simulink model "TDE_with_NPD_ARAS"  (R2018b)
settings: Solver=FixedStepAuto  StartTime=0.0  StopTime=24.5  FixedStep=.001  RelTol=1e-3
settings Model: Creator=ahmad  LastModifiedBy=asus
settings SFSimCC: SimUseLocalCustomCode=off
settings RTWCC: RTWUseLocalCustomCode=off
settings CodeAppCC: StateflowObjectComments=on

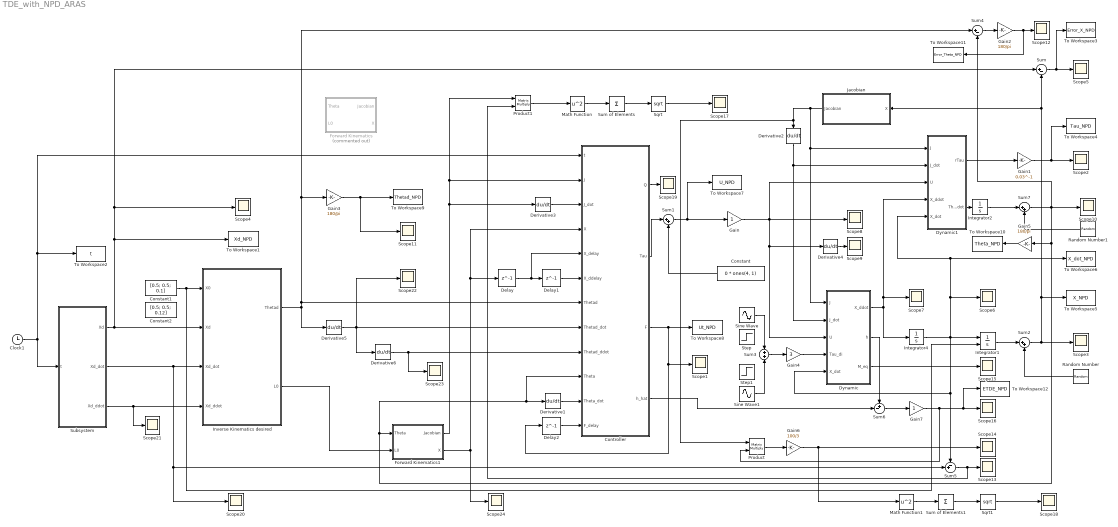
== system TDE_with_NPD_ARAS ==
  Clock1 : Clock
  Constant : Constant  Value=0 * ones(4, 1)
  Constant1 : Constant  Value=[0.5; 0.5; 0.1]
  Constant2 : Constant  Value=[0.5; 0.5; 0.12]
  "Controller " : MATLAB Function  TreatAsAtomicUnit=on
  Delay : Delay  DelayLength=1  InitialCondition=[0; 0; 0]
  Delay1 : Delay  DelayLength=1  InitialCondition=[0; 0; 0]
  Delay2 : Delay  DelayLength=1  InitialCondition=[0; 0; 0]
  Derivative{1..6} (6 alike) : Derivative
  Dynamic : MATLAB Function  TreatAsAtomicUnit=on
  Dynamic1 : MATLAB Function  TreatAsAtomicUnit=on
  Forward Kinematics : MATLAB Function  Commented=on  TreatAsAtomicUnit=on
  Forward Kinematics1 : MATLAB Function  TreatAsAtomicUnit=on
  Gain : Gain
  Gain1 : Gain  Gain=0.03^-1
  Gain2 : Gain  Gain=180/pi
  Gain3 : Gain  Gain=180/pi
  Gain4 : Gain  Gain=3
  Gain5 : Gain  Gain=180/pi
  Gain6 : Gain  Gain=100/3
  Gain7 : Gain
  Integrator1 : Integrator  InitialConditionSource=external  InitialCondition=[0.5; 0.5; 0.5]
  Integrator2 : Integrator  InitialCondition=[0;0;0;0]
  Integrator4 : Integrator  InitialCondition=[0;0;0]
  Inverse Kinematics desired : MATLAB Function  TreatAsAtomicUnit=on
  Jacobian : MATLAB Function  TreatAsAtomicUnit=on
  Math Function : Math  Operator=square  SaturateOnIntegerOverflow=on
  Math Function1 : Math  Operator=square  SaturateOnIntegerOverflow=on
  Product : Product  Multiplication=Matrix(*)
  Product1 : Product  Multiplication=Matrix(*)
  Random Number : RandomNumber  Mean=[0;0;0]  Variance=0.0000 * ones(3, 1)  SampleTime=0.01
  Random Number1 : RandomNumber  Mean=[0;0;0;0]  Variance=0.0000 * ones(4, 1)  SampleTime=0.01
  Scope{1..24} (24 alike) : Scope
  Sine Wave : Sin  Phase=pi/2
  Sine Wave1 : Sin  Amplitude=0
  Sqrt : Sqrt  SaturateOnIntegerOverflow=on
  Sqrt1 : Sqrt  SaturateOnIntegerOverflow=on
  Step : Step  Time=15  Before=[0; 0; 0]  After=[-1; 1; 1]  SampleTime=0.001
  Step1 : Step  Time=17  Before=[0; 0; 0]  After=[1; -1; -1]  SampleTime=0.001
  Subsystem : Subsystem
  Sum : Sum  Inputs=|+-
  Sum of Elements : Sum  Inputs=+
  Sum of Elements1 : Sum  Inputs=+
  Sum1 : Sum  Inputs=|++
  Sum2 : Sum  Inputs=|++
  Sum3 : Sum
  Sum4 : Sum  Inputs=|+-
  Sum5 : Sum  Inputs=-+|
  Sum6 : Sum  Inputs=+-|
  Sum7 : Sum  Inputs=|++
  To Workspace1 : ToWorkspace  VariableName=Xd_NPD  SampleTime=-1
  To Workspace10 : ToWorkspace  VariableName=Theta_NPD  SampleTime=-1
  To Workspace11 : ToWorkspace  VariableName=Error_Theta_NPD  SampleTime=-1
  To Workspace12 : ToWorkspace  VariableName=ETDE_NPD  SampleTime=-1
  To Workspace2 : ToWorkspace  VariableName=t  SampleTime=-1
  To Workspace3 : ToWorkspace  VariableName=Error_X_NPD  SampleTime=-1
  To Workspace4 : ToWorkspace  VariableName=Tau_NPD  SampleTime=-1
  To Workspace5 : ToWorkspace  VariableName=X_NPD  SampleTime=-1
  To Workspace6 : ToWorkspace  VariableName=X_dot_NPD  SampleTime=-1
  To Workspace7 : ToWorkspace  VariableName=U_NPD  SampleTime=-1
  To Workspace8 : ToWorkspace  VariableName=Ut_NPD  SampleTime=-1
  To Workspace9 : ToWorkspace  VariableName=Thetad_NPD  SampleTime=-1
  wires:
  Integrator1/1 -> Sum2/1
  Sum/1 -> To Workspace3/1, Scope5/1
  Constant/1 -> Sum1/2
  Random Number/1 -> Sum2/2
  Sum2/1 -> To Workspace5/1, Jacobian/1(X), Sum/2, Scope3/1
  Clock1/1 -> To Workspace2/1, "Controller "/1(t), Subsystem/1(t)
  Delay/1 -> "Controller "/5(X_delay), Delay1/1
  Delay1/1 -> "Controller "/6(X_ddelay)
  "Controller "/3(F) -> Delay2/1, Scope1/1, To Workspace8/1
  "Controller "/2(Tau) -> Sum1/1
  Delay2/1 -> "Controller "/12(F_delay)
  Sum1/1 -> Gain/1, To Workspace7/1
  Inverse Kinematics desired/1(Thetad) -> Derivative5/1, Gain3/1, Sum4/1, "Controller "/7(Thetad)
  Derivative1/1 -> "Controller "/11(Theta_dot)
  Sum3/1 -> Gain4/1
  Sine Wave/1 -> Sum3/1
  Sine Wave1/1 -> Sum3/2
  Gain1/1 -> To Workspace4/1, Scope2/1
  Dynamic/1(X_ddot) -> Integrator4/1, Dynamic1/4(X_ddot), Scope7/1
  Jacobian/1(Jacobian) -> Product/1, Derivative2/1, Dynamic1/1(J), Dynamic/1(J)
  Derivative3/1 -> "Controller "/3(J_dot)
  Integrator4/1 -> To Workspace6/1, Dynamic1/5(X_dot), Scope6/1, Sum5/1, Dynamic/5(X_dot), Integrator1/1
  Dynamic1/1(rTau) -> Gain1/1
  Gain/1 -> Derivative4/1, Dynamic/3(U), Scope8/1, Dynamic1/3(U)
  Forward Kinematics1/1(Jacobian) -> Product1/1, "Controller "/2(J), Derivative3/1
  Forward Kinematics1/2(X) -> "Controller "/4(X), Delay/1, Scope24/1
  Derivative2/1 -> Dynamic/2(J_dot), Dynamic1/2(J_dot)
  Subsystem/1(Xd) -> Inverse Kinematics desired/2(Xd), To Workspace1/1, Scope4/1, Sum/1
  Subsystem/2(Xd_dot) -> Scope20/1, Sum5/2, Inverse Kinematics desired/3(Xd_dot)
  Subsystem/3(Xd_ddot) -> Scope21/1, Inverse Kinematics desired/4(Xd_ddot)
  Derivative4/1 -> Scope9/1
  Dynamic1/2(Theta_dot) -> Integrator2/1
  Sum7/1 -> Sum4/2, Forward Kinematics1/1(Theta), "Controller "/10(Theta), Derivative1/1, Gain5/1, Scope10/1
  Sum4/1 -> Gain2/1
  Gain2/1 -> To Workspace11/1, Scope12/1
  Gain3/1 -> Scope11/1, To Workspace9/1
  Gain4/1 -> Dynamic/4(Tau_di)
  Gain5/1 -> To Workspace10/1
  Dynamic/2(h) -> Sum6/1
  "Controller "/4(h_hat) -> Sum6/2
  Sum6/1 -> Gain7/1
  Product/1 -> Gain6/1
  Dynamic/3(M_eq) -> Scope15/1
  Sum of Elements/1 -> Sqrt/1
  Math Function/1 -> Sum of Elements/1
  Sum5/1 -> Product1/2, Scope13/1
  Product1/1 -> Math Function/1
  Sqrt/1 -> Scope17/1
  Gain6/1 -> Math Function1/1, Scope14/1
  Sqrt1/1 -> Scope18/1
  Math Function1/1 -> Sum of Elements1/1
  Sum of Elements1/1 -> Sqrt1/1
  Integrator2/1 -> Sum7/1
  Random Number1/1 -> Sum7/2
  "Controller "/1(Q) -> Scope19/1
  Constant1/1 -> Inverse Kinematics desired/1(X0), Integrator1/2
  Derivative5/1 -> Derivative6/1, Scope22/1, "Controller "/8(Thetad_dot)
  Derivative6/1 -> Scope23/1, "Controller "/9(Thetad_ddot)
  Inverse Kinematics desired/2(L0) -> Forward Kinematics1/2(L0)
  Gain7/1 -> Product/2, To Workspace12/1, Scope16/1

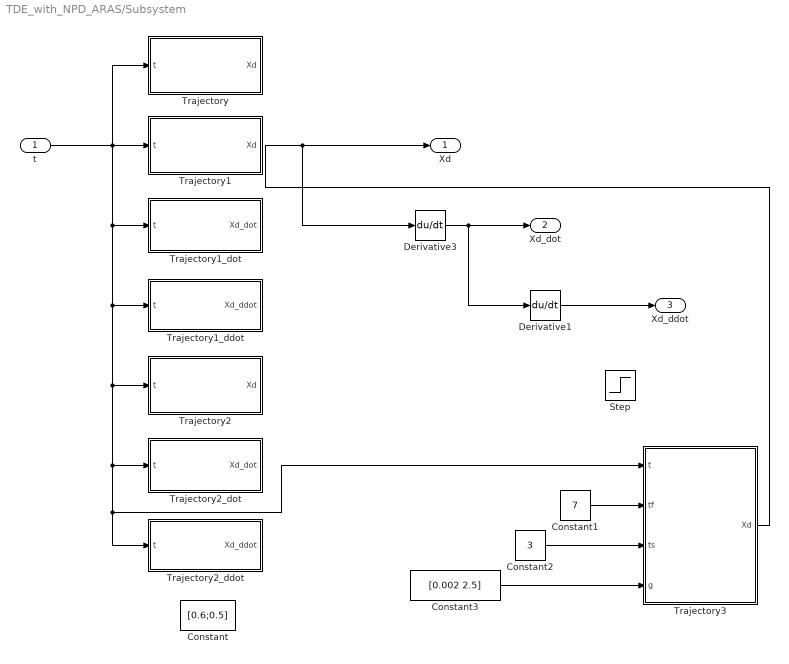
== system TDE_with_NPD_ARAS/Subsystem ==
  t : Inport
  Constant : Constant  Value=[0.6;0.5]
  Constant1 : Constant  Value=7
  Constant2 : Constant  Value=3
  Constant3 : Constant  Value=[0.002 2.5]
  Derivative1 : Derivative
  Derivative3 : Derivative
  Step : Step  Time=10  Before=[0.5; 0.5; 0.1]  After=[0.5; 0.5; 0.13]  SampleTime=0.001
  Trajectory : MATLAB Function  TreatAsAtomicUnit=on
  Trajectory1 : MATLAB Function  TreatAsAtomicUnit=on
  Trajectory1_ddot : MATLAB Function  TreatAsAtomicUnit=on
  Trajectory1_dot : MATLAB Function  TreatAsAtomicUnit=on
  Trajectory2 : MATLAB Function  TreatAsAtomicUnit=on
  Trajectory2_ddot : MATLAB Function  TreatAsAtomicUnit=on
  Trajectory2_dot : MATLAB Function  TreatAsAtomicUnit=on
  Trajectory3 : MATLAB Function  TreatAsAtomicUnit=on
  Xd : Outport
  Xd_dot : Outport  Port=2
  Xd_ddot : Outport  Port=3
  wires:
  Trajectory3/1(Xd) -> Derivative3/1, Xd/1
  Derivative3/1 -> Derivative1/1, Xd_dot/1
  Derivative1/1 -> Xd_ddot/1
  Constant2/1 -> Trajectory3/3(ts)
  Constant3/1 -> Trajectory3/4(g)
  Constant1/1 -> Trajectory3/2(tf)
  t/1 -> Trajectory/1(t), Trajectory3/1(t), Trajectory2_ddot/1(t), Trajectory2_dot/1(t), Trajectory2/1(t), Trajectory1_ddot/1(t), Trajectory1_dot/1(t), Trajectory1/1(t)

== matlab function TDE_with_NPD_ARAS/Dynamic ==
  data: J input; J_dot input; U input; Tau_di input; X_ddot output; X_dot input; h output; M_eq output
function [X_ddot, h, M_eq] = fcn(J, J_dot, U, Tau_di, X_dot)

M_bar = 0.01 * eye(3);
m = 1.5;
g = 9.81;
r = 0.03;

Im = 8.31 * 10^-5 * eye(4);
Dm = 2.16 * 10^-4 * eye(4);

M = m * eye(3);
C = zeros(3, 3);
G = [0; 0; m*g];
N = C * X_dot + G + 0.5 * sign(X_dot) + 0.5 * X_dot + Tau_di;

M_eq = r * M + r^-1 * J' * Im * J;
N_eq = r * N + r^-1 * J' * Im * J_dot * X_dot + r^-1 * J' * Dm * J * X_dot;
% W = J';
Tau = J' * U;
X_ddot = M_eq^(-1) * (Tau - N_eq);
h = (M_eq - M_bar) * X_ddot + N_eq;
end

== matlab function TDE_with_NPD_ARAS/Dynamic1 ==
  data: J input; rTau output; J_dot input; U input; X_ddot input; X_dot input; Theta_dot output
function [rTau, Theta_dot] = fcn(J, J_dot, U, X_ddot, X_dot)

r = 0.03;
Im = 8.31 * 10^-5 * eye(4);
Dm = 2.16 * 10^-4 * eye(4);

Theta_dot = r^-1 * J * X_dot;
Theta_ddot = r^-1 * (J * X_ddot + J_dot * X_dot);

rTau = Im * Theta_ddot + Dm * Theta_dot - U;
end

== matlab function TDE_with_NPD_ARAS/Subsystem/Trajectory1 ==
  data: Xd output; t input
function Xd = fcn(t)

a = 1.00;
b = 1.00;
r = 0.1;
f = 0.5;

x = r * (cos(2*pi*f*t)) + a/2;
y = r * (sin(2*pi*f*t)) + b/2;

Xd = [x y]';
end

== matlab function TDE_with_NPD_ARAS/Inverse Kinematics desired ==
  data: X0 input; Xd input; Thetad output; Xd_dot input; Xd_ddot input; L0 output
function [Thetad, L0]  = fcn(X0, Xd, Xd_dot, Xd_ddot)

a = 1.00;% + 0.05;
b = 1.00;% - 0.05;
c = 1.00;% - 0.05;
r = 0.03;

% A1 = [0+0.02 0-0.01 c-0.1]';
% A2 = [0+0.01 b+0.01 c+0.1]';
% A3 = [a-0.02 b-0.02 c-0.02]';
% A4 = [a-0.01 0+0.02 c+0.02]';
A1 = [0 0 c]';
A2 = [0 b c]';
A3 = [a b c]';
A4 = [a 0 c]';

L0 = [sqrt((X0(1)-A1(1))^2 + (X0(2)-A1(2))^2 + (X0(3)-A1(3))^2)
      sqrt((X0(1)-A2(1))^2 + (X0(2)-A2(2))^2 + (X0(3)-A2(3))^2)
      sqrt((X0(1)-A3(1))^2 + (X0(2)-A3(2))^2 + (X0(3)-A3(3))^2)
      sqrt((X0(1)-A4(1))^2 + (X0(2)-A4(2))^2 + (X0(3)-A4(3))^2)];

L = [sqrt((Xd(1)-A1(1))^2 + (Xd(2)-A1(2))^2 + (Xd(3)-A1(3))^2)
     sqrt((Xd(1)-A2(1))^2 + (Xd(2)-A2(2))^2 + (Xd(3)-A2(3))^2)
     sqrt((Xd(1)-A3(1))^2 + (Xd(2)-A3(2))^2 + (Xd(3)-A3(3))^2)
     sqrt((Xd(1)-A4(1))^2 + (Xd(2)-A4(2))^2 + (Xd(3)-A4(3))^2)];
 
Thetad = r^-1 * (L - L0);
end

== matlab function TDE_with_NPD_ARAS/Forward Kinematics ==
  data: Jacobian output; Theta input; X output; L0 input
function [Jacobian, X] = fcn(Theta, L0)

a = 1.00;% + 0.05;
b = 1.00;% - 0.05;
c = 1.00;% - 0.05;
r = 0.03;% + 0.005;

A1 = [0 0 c]';
A2 = [0 b c]';
A3 = [a b c]';
A4 = [a 0 c]';
% A1 = [0+0.02 0-0.01 c-0.1]';
% A2 = [0+0.01 b+0.01 c+0.1]';
% A3 = [a-0.02 b-0.02 c-0.02]';
% A4 = [a-0.01 0+0.02 c+0.02]';

L = [r * Theta(1) + L0(1)
     r * Theta(2) + L0(2)
     r * Theta(3) + L0(3)
     r * Theta(4) + L0(4)];
% dgfd
g1 = A1(1)^2-A2(1)^2+A1(2)^2-A2(2)^2+A1(3)^2-A2(3)^2;
g2 = A1(1)^2-A3(1)^2+A1(2)^2-A3(2)^2+A1(3)^2-A3(3)^2;

e1 = (L(1)^2-L(2)^2-g1) / (2*(A2(2)-A1(2)));
e2 = (A2(1)-A1(1)) / (A2(2)-A1(2));
e3 = (A2(3)*A1(3)) / (A2(2)-A1(2));
f1 = (L(1)^2-L(3)^2-g2) / (2*(A3(1)-A1(1)));
f2 = (A3(2)-A1(2)) / (A3(1)-A1(1));
f3 = (A3(3)-A1(3)) / (A3(1)-A1(1));

d1 = (e1-e2*f1) / (1-e2*f2);
d2 = (e3-e2*f3) / (1-e2*f2);
d3 = f1-f2*d1;
d4 = f2*d2-f3;

A = 1 + d2^2 + d4^2;
B = 2*(d3*d4-A1(1)*d4-d1*d2+A1(2)*d2-A1(3));
C = d3^2+A1(1)^2-2*A1(1)*d3+d1^2+A1(2)^2-2*A1(2)*d1+A1(3)^2-L(1)^2;

z = (-B-sqrt(B^2-4*A*C)) / (2*A);
y = d1 - d2 * z;
x = d3 + d4 * z;
% x = (L(2)^2 - L(3)^2 + a^2) / (2*a);
% y = (L(1)^2 - L(2)^2 + b^2) / (2*b);
% z = c - sqrt(L(1)^2 - x^2 - y^2);
X = [x y z]';

Jacobian = [(X(1)-A1(1))/L(1)    (X(2)-A1(2))/L(1)   (X(3)-A1(3))/L(1)
            (X(1)-A2(1))/L(2)    (X(2)-A2(2))/L(2)   (X(3)-A2(3))/L(2)
            (X(1)-A3(1))/L(3)    (X(2)-A3(2))/L(3)   (X(3)-A3(3))/L(3)
            (X(1)-A4(1))/L(4)    (X(2)-A4(2))/L(4)   (X(3)-A4(3))/L(4)];
end

== matlab function TDE_with_NPD_ARAS/Subsystem/Trajectory ==
  data: Xd output; t input
function Xd  = fcn(t)

a = 1.00;
b = 1.00;
ts = 2;
tf = 5;

if t <= ts
    x0 = a / 2;
    y0 = b / 2;
    Xd = [x0 y0]';
elseif t > ts && t < tf+ts
    x0 = a / 2; xf = x0 - 0.0; x_dot0 = 0; x_dotf = 0; x_ddot0 = 0; x_ddotf = 0;
    a0 = x0; a1 = x_dot0; a2 = x_ddot0 / 2;
    a3 = (20*(xf-x0)-(8*x_dotf+12*x_dot0)*tf-(3*x_ddot0-x_ddotf)*tf^2) / (2*tf^3);
    a4 = (30*(x0-xf)+(14*x_dotf+16*x_dot0)*tf+(3*x_ddot0-2*x_ddotf)*tf^2) / (2*tf^4);
    a5 = (12*(xf-x0)-(6*x_dotf+6*x_dot0)*tf-(x_ddot0-x_ddotf)*tf^2) / (2*tf^5);
    x = a0 + a1 * (t-ts) + a2 * (t-ts)^2 + a3 * (t-ts)^3 + a4 * (t-ts)^4 + a5 * (t-ts)^5;
    
    y0 = b / 2; yf = y0 + 0.2; y_dot0 = 0; y_dotf = 0; y_ddot0 = 0; y_ddotf = 0;
    b0 = y0; b1 = y_dot0; b2 = y_ddot0 / 2;
    b3 = (20*(yf-y0)-(8*y_dotf+12*y_dot0)*tf-(3*y_ddot0-y_ddotf)*tf^2) / (2*tf^3);
    b4 = (30*(y0-yf)+(14*y_dotf+16*y_dot0)*tf+(3*y_ddot0-2*y_ddotf)*tf^2) / (2*tf^4);
    b5 = (12*(yf-y0)-(6*y_dotf+6*y_dot0)*tf-(y_ddot0-y_ddotf)*tf^2) / (2*tf^5);
    y = b0 + b1 * (t-ts) + b2 * (t-ts)^2 + b3 * (t-ts)^3 + b4 * (t-ts)^4 + b5 * (t-ts)^5;
    
    Xd = [x y]';
elseif t >= tf+ts && t < 10
    x0 = a / 2; xf = x0 - 0.0;
    y0 = b / 2; yf = y0 + 0.2;
    
    Xd = [xf yf]';
elseif t >= 10 && t < 30
    f = 0.05;
    x = 0.5 + 0.2*sin(2*pi*f*(t-10));
    y = 0.5 + 0.2*cos(2*pi*f*(t-10));

    Xd = [x y]';
elseif t >= 30 && t < 40
    f = 0.1;
    x = 0.5 + 0.2*sin(2*pi*f*(t-30));
    y = 0.5 + 0.2*cos(2*pi*f*(t-30));

    Xd = [x y]';
elseif t >= 40 && t < 45
    f = 0.2;
    x = 0.5 + 0.2*sin(2*pi*f*(t-40));
    y = 0.5 + 0.2*cos(2*pi*f*(t-40));

    Xd = [x y]';
elseif t >= 45 && t < 47
    f = 0.5;
    x = 0.5 + 0.2*sin(2*pi*f*(t-45));
    y = 0.5 + 0.2*cos(2*pi*f*(t-45));

    Xd = [x y]';
elseif t >= 47 && t < 49
    f = 0.5;
    x = 0.5 + 0.2*sin(2*pi*f*(t-47));
    y = 0.5 + 0.2*cos(2*pi*f*(t-47));

    Xd = [x y]';
elseif t >= 49 && t < 54
    f = 0.2;
    x = 0.5 + 0.2*sin(2*pi*f*(t-49));
    y = 0.5 + 0.2*cos(2*pi*f*(t-49));

    Xd = [x y]';
elseif t >= 54 && t < 64
    f = 0.1;
    x = 0.5 + 0.2*sin(2*pi*f*(t-54));
    y = 0.5 + 0.2*cos(2*pi*f*(t-54));

    Xd = [x y]';
elseif t >= 64 && t < 84
    f = 0.05;
    x = 0.5 + 0.2*sin(2*pi*f*(t-64));
    y = 0.5 + 0.2*cos(2*pi*f*(t-64));

    Xd = [x y]';
elseif t >= 84 && t < tf+84
    x0 = a / 2; xf = x0 - 0.0; x_dot0 = 0; x_dotf = 0; x_ddot0 = 0; x_ddotf = 0;
    a0 = x0; a1 = x_dot0; a2 = x_ddot0 / 2;
    a3 = (20*(xf-x0)-(8*x_dotf+12*x_dot0)*tf-(3*x_ddot0-x_ddotf)*tf^2) / (2*tf^3);
    a4 = (30*(x0-xf)+(14*x_dotf+16*x_dot0)*tf+(3*x_ddot0-2*x_ddotf)*tf^2) / (2*tf^4);
    a5 = (12*(xf-x0)-(6*x_dotf+6*x_dot0)*tf-(x_ddot0-x_ddotf)*tf^2) / (2*tf^5);
    x = a0 + a1 * (t-84) + a2 * (t-84)^2 + a3 * (t-84)^3 + a4 * (t-84)^4 + a5 * (t-84)^5;
    
    y0 = b / 2 + 0.2; yf = y0 - 0.2; y_dot0 = 0; y_dotf = 0; y_ddot0 = 0; y_ddotf = 0;
    b0 = y0; b1 = y_dot0; b2 = y_ddot0 / 2;
    b3 = (20*(yf-y0)-(8*y_dotf+12*y_dot0)*tf-(3*y_ddot0-y_ddotf)*tf^2) / (2*tf^3);
    b4 = (30*(y0-yf)+(14*y_dotf+16*y_dot0)*tf+(3*y_ddot0-2*y_ddotf)*tf^2) / (2*tf^4);
    b5 = (12*(yf-y0)-(6*y_dotf+6*y_dot0)*tf-(y_ddot0-y_ddotf)*tf^2) / (2*tf^5);
    y = b0 + b1 * (t-84) + b2 * (t-84)^2 + b3 * (t-84)^3 + b4 * (t-84)^4 + b5 * (t-84)^5;
    
    Xd = [x y]';
else
    x0 = a / 2;
    y0 = b / 2;
    xf = x0 + 0.0;
    yf = y0 + 0.0;
    Xd = [xf yf]';
end

end

== matlab function TDE_with_NPD_ARAS/Subsystem/Trajectory2 ==
  data: Xd output; t input
function Xd = fcn(t)

T = 0.001;
a = 1;
b = 1;

x0 = b / 2 - 0.1; xf = x0 + 0.3; x_dot0 = 0; x_dotf = 0; tf = 10;
a0 = x0; a1 = x_dot0; a2 = (3/tf^2) * (xf-x0) - ((x_dotf+2*x_dot0) / tf); a3 = (-2/tf^3) * (xf-x0) + (x_dotf+x_dot0) / tf^2;
x = a0 + a1 * t + a2 * t^2 + a3 * t^3;
x_new = a0 + a1 * (t + T) + a2 * (t + T)^2 + a3 * (t + T)^3;

y0 = a / 2 - 0.1; yf = y0 + 0.3; y_dot0 = 0; y_dotf = 0;
b0 = y0; b1 = y_dot0; b2 = (3/tf^2) * (yf-y0) - ((y_dotf+2*y_dot0) / tf); b3 = (-2/tf^3) * (yf-y0) + (y_dotf+y_dot0) / tf^2;
y = b0 + b1 * t + b2 * t^2 + b3 * t^3;
y_new = b0 + b1 * (t + T) + b2 * (t + T)^2 + b3 * (t + T)^3;

Xd = [x y]';
Xr_new = [x_new y_new]';
end

== matlab function TDE_with_NPD_ARAS/Jacobian ==
  data: Jacobian output; X input
function Jacobian = fcn(X)

a = 1.00;
b = 1.00;
c = 1.00;
% r = 0.03;

L = [sqrt((X(1)-0)^2 + (X(2)-0)^2 + (X(3)-c)^2)
     sqrt((X(1)-0)^2 + (X(2)-b)^2 + (X(3)-c)^2)
     sqrt((X(1)-a)^2 + (X(2)-b)^2 + (X(3)-c)^2)
     sqrt((X(1)-a)^2 + (X(2)-0)^2 + (X(3)-c)^2)];

Jacobian = [(X(1)-0)/L(1)    (X(2)-0)/L(1)   (X(3)-c)/L(1)
            (X(1)-0)/L(2)    (X(2)-b)/L(2)   (X(3)-c)/L(2)
            (X(1)-a)/L(3)    (X(2)-b)/L(3)   (X(3)-c)/L(3)
            (X(1)-a)/L(4)    (X(2)-0)/L(4)   (X(3)-c)/L(4)];
end

== matlab function TDE_with_NPD_ARAS/Controller  ==
  settings: updateMethod=DISCRETE
  data: Q output; t input; Tau output; J input; J_dot input; X input; X_delay input; X_ddelay input; Thetad input; Thetad_dot input; Thetad_ddot input; Theta input; Theta_dot input; F_delay input; F output; h_hat output
function [Q, Tau, F, h_hat] = fcn(t, J, J_dot, X, X_delay, X_ddelay, Thetad, Thetad_dot, Thetad_ddot, Theta, Theta_dot, F_delay)

T = 0.001;
r = 0.03 ;%+ 0.005;
Q = zeros(4, 1);
k = -2;
% tau_min = [0.01 0.01 0.01]';
% tau_max = [1.5 1.5 1.5]';

deltap = 5 * 10^-4;
deltav = 5 * 10^-4;
alphap = 0.3;
alphav = 1.4;
M_bar = 0.01 * eye(3);
Kp = 25 * eye(4);
Kv = 2 * Kp.^0.5;
Ke = 10 * eye(4);

Error = Thetad - Theta;
Error_dot = Thetad_dot - Theta_dot;

if norm(Error) > deltap
    N_Kp = Kp * diag((abs(Error)).^(alphap - 1));
else
    N_Kp = diag([deltap.^(alphap - 1), deltap.^(alphap - 1), deltap.^(alphap - 1), deltap.^(alphap - 1)]);
end

if norm(Error_dot) > deltav
    N_Kv = Kv * diag((abs(Error_dot)).^(alphav - 1));
else
    N_Kv = diag([deltav.^(alphav - 1), deltav.^(alphav - 1), deltav.^(alphav - 1), deltav.^(alphav - 1)]);
end

if t <= 2*T
    X_ddot_delay = zeros(3, 1);
else
    X_ddot_delay = (X - 2 * X_delay + X_ddelay) / T^2;
end

h_hat = F_delay - M_bar * X_ddot_delay;

W = J';
Ur = M_bar * (r * pinv(J) * (Thetad_ddot + N_Kv * Error_dot + N_Kp * Error - J_dot * pinv(J) * Theta_dot + Ke * sat(Error_dot))) + h_hat;
Tau = pinv(W) * Ur; % + k * null(W);
Q = pinv(W) * Ur + k * null(W) - pinv(W) * Ur;
F = W * Tau;
end

function S = sat(E_dot)

varpi = 0.10;

if norm(E_dot) >= varpi
     S = E_dot / norm(E_dot);
else
    S = E_dot / varpi;
end
end

== matlab function TDE_with_NPD_ARAS/Subsystem/Trajectory1_ddot ==
  data: Xd_ddot output; t input
function Xd_ddot = fcn(t)

a = 1.00;
b = 1.00;
r = 0.1;
f = 0.5;

x_ddot = -r * ((2*pi*f)^2*cos(2*pi*f*t));
y_ddot = -r * ((2*pi*f)^2*sin(2*pi*f*t));

Xd_ddot = [x_ddot y_ddot]';
end

== matlab function TDE_with_NPD_ARAS/Subsystem/Trajectory1_dot ==
  data: Xd_dot output; t input
function Xd_dot = fcn(t)

a = 1.00;
b = 1.00;
r = 0.1;
f = 0.5;

x_dot = -r * (2*pi*f*sin(2*pi*f*t));
y_dot = +r * (2*pi*f*cos(2*pi*f*t));

Xd_dot = [x_dot y_dot]';
end

== matlab function TDE_with_NPD_ARAS/Subsystem/Trajectory2_ddot ==
  data: Xd_ddot output; t input
function Xd_ddot = fcn(t)

T = 0.001;
a = 1;
b = 1;

x0 = b / 2 - 0.1; xf = x0 + 0.3; x_dot0 = 0; x_dotf = 0; tf = 10;
a2 = (3/tf^2) * (xf-x0) - ((x_dotf+2*x_dot0) / tf); a3 = (-2/tf^3) * (xf-x0) + (x_dotf+x_dot0) / tf^2;
x_ddot = 2 * a2 + 6 * a3 * t;
x_ddot_new = 2 * a2 + 6 * a3 * (t + T);

y0 = a / 2 - 0.1; yf = y0 + 0.3; y_dot0 = 0; y_dotf = 0;
b2 = (3/tf^2) * (yf-y0) - ((y_dotf+2*y_dot0) / tf); b3 = (-2/tf^3) * (yf-y0) + (y_dotf+y_dot0) / tf^2;
y_ddot = 2 * b2 + 6 * b3 * t;
y_ddot_new = 2 * b2 + 6 * b3 * (t + T);

Xd_ddot = [x_ddot y_ddot]';
Xr_ddot_new = [x_ddot_new y_ddot_new]';
end

== matlab function TDE_with_NPD_ARAS/Subsystem/Trajectory2_dot ==
  data: Xd_dot output; t input
function Xd_dot = fcn(t)

T = 0.001;
a = 1;
b = 1;

x0 = b / 2 - 0.1; xf = x0 + 0.3; x_dot0 = 0; x_dotf = 0; tf = 10;
a1 = x_dot0; a2 = (3/tf^2) * (xf-x0) - ((x_dotf+2*x_dot0) / tf); a3 = (-2/tf^3) * (xf-x0) + (x_dotf+x_dot0) / tf^2;
x_dot = a1 + 2 * a2 * t + 3 * a3 * t^2;
x_dot_new = a1 + 2 * a2 * (t + T) + 3 * a3 * (t + T)^2;


y0 = a / 2 - 0.1; yf = y0 + 0.3; y_dot0 = 0; y_dotf = 0;
b1 = y_dot0; b2 = (3/tf^2) * (yf-y0) - ((y_dotf+2*y_dot0) / tf); b3 = (-2/tf^3) * (yf-y0) + (y_dotf+y_dot0) / tf^2;
y_dot = b1 + 2 * b2 * t + 3 * b3 * t^2;
y_dot_new = b1 + 2 * b2 * (t + T) + 3 * b3 * (t + T)^2;

Xd_dot = [x_dot y_dot]';
Xr_dot_new = [x_dot_new y_dot_new]';

end

== matlab function TDE_with_NPD_ARAS/Subsystem/Trajectory3 ==
  settings: updateMethod=DISCRETE
  data: Xd output; t input; tf input; ts input; g input
function Xd = fcn(t, tf, ts, g)

persistent phi
if isempty(phi)
    phi = 0;
end
x0 = 0.5;
y0 = 0.5;
z0 = 0.1;
if t < ts
    x = x0;
    y = y0;
    z = z0;
    
    Xd = [x y z]';
elseif t >= ts && t < ts+tf
    xf = x0 + 0.0; x_dot0 = 0; x_dotf = 0; x_ddot0 = 0; x_ddotf = 0;
    a0 = x0; a1 = x_dot0; a2 = x_ddot0 / 2;
    a3 = (20*(xf-x0)-(8*x_dotf+12*x_dot0)*tf-(3*x_ddot0-x_ddotf)*tf^2) / (2*tf^3);
    a4 = (30*(x0-xf)+(14*x_dotf+16*x_dot0)*tf+(3*x_ddot0-2*x_ddotf)*tf^2) / (2*tf^4);
    a5 = (12*(xf-x0)-(6*x_dotf+6*x_dot0)*tf-(x_ddot0-x_ddotf)*tf^2) / (2*tf^5);
    x = a0 + a1 * (t-ts) + a2 * (t-ts)^2 + a3 * (t-ts)^3 + a4 * (t-ts)^4 + a5 * (t-ts)^5;
    
    yf = y0 + 0.1; y_dot0 = 0; y_dotf = 0; y_ddot0 = 0; y_ddotf = 0;
    b0 = y0; b1 = y_dot0; b2 = y_ddot0 / 2;
    b3 = (20*(yf-y0)-(8*y_dotf+12*y_dot0)*tf-(3*y_ddot0-y_ddotf)*tf^2) / (2*tf^3);
    b4 = (30*(y0-yf)+(14*y_dotf+16*y_dot0)*tf+(3*y_ddot0-2*y_ddotf)*tf^2) / (2*tf^4);
    b5 = (12*(yf-y0)-(6*y_dotf+6*y_dot0)*tf-(y_ddot0-y_ddotf)*tf^2) / (2*tf^5);
    y = b0 + b1 * (t-ts) + b2 * (t-ts)^2 + b3 * (t-ts)^3 + b4 * (t-ts)^4 + b5 * (t-ts)^5;

    zf = z0 + 0.4; z_dot0 = 0; z_dotf = 0; z_ddot0 = 0; z_ddotf = 0;
    c0 = z0; c1 = z_dot0; c2 = z_ddot0 / 2;
    c3 = (20*(zf-z0)-(8*z_dotf+12*z_dot0)*tf-(3*z_ddot0-z_ddotf)*tf^2) / (2*tf^3);
    c4 = (30*(z0-zf)+(14*z_dotf+16*z_dot0)*tf+(3*z_ddot0-2*z_ddotf)*tf^2) / (2*tf^4);
    c5 = (12*(zf-z0)-(6*z_dotf+6*z_dot0)*tf-(z_ddot0-z_ddotf)*tf^2) / (2*tf^5);
    z = c0 + c1 * (t-ts) + c2 * (t-ts)^2 + c3 * (t-ts)^3 + c4 * (t-ts)^4 + c5 * (t-ts)^5;
    
    Xd = [x y z]';
elseif (t >= ts+tf && t < 30)
    phi = phi + g(1)*0.5*(1+tanh(1.5*(t-12)))*pi/g(2);
    x = 0.5 + 0.1*sin(phi);
    y = 0.5 + 0.1*cos(phi);
    z = z0 + 0.4;
    
    Xd = [x y z]';
elseif (t >= 30 && t < 35)
    phi = phi + g(1)*0.5*(1-tanh(1.5*(t-32)))*pi/g(2);
    x = 0.5 + 0.1*sin(phi);
    y = 0.5 + 0.1*cos(phi);
    z = z0 + 0.4;
    
    Xd = [x y z]';
elseif (t >= 35 && t < 40)
    x = 0.5 + 0.1*sin(phi);
    y = 0.5 + 0.1*cos(phi);
    z = z0 + 0.4;
    
    Xd = [x y z]';
elseif (t >= 40 && t < 40+tf)
    x0 = 0.5 + 0.1*sin(phi); xf = x0 - 0.0; x_dot0 = 0; x_dotf = 0; x_ddot0 = 0; x_ddotf = 0;
    a0 = x0; a1 = x_dot0; a2 = x_ddot0 / 2;
    a3 = (20*(xf-x0)-(8*x_dotf+12*x_dot0)*tf-(3*x_ddot0-x_ddotf)*tf^2) / (2*tf^3);
    a4 = (30*(x0-xf)+(14*x_dotf+16*x_dot0)*tf+(3*x_ddot0-2*x_ddotf)*tf^2) / (2*tf^4);
    a5 = (12*(xf-x0)-(6*x_dotf+6*x_dot0)*tf-(x_ddot0-x_ddotf)*tf^2) / (2*tf^5);
    x = a0 + a1 * (t-40) + a2 * (t-40)^2 + a3 * (t-40)^3 + a4 * (t-40)^4 + a5 * (t-40)^5;
    
    y0 = 0.5 + 0.1*cos(phi); yf = y0 - 0.1; y_dot0 = 0; y_dotf = 0; y_ddot0 = 0; y_ddotf = 0;
    b0 = y0; b1 = y_dot0; b2 = y_ddot0 / 2;
    b3 = (20*(yf-y0)-(8*y_dotf+12*y_dot0)*tf-(3*y_ddot0-y_ddotf)*tf^2) / (2*tf^3);
    b4 = (30*(y0-yf)+(14*y_dotf+16*y_dot0)*tf+(3*y_ddot0-2*y_ddotf)*tf^2) / (2*tf^4);
    b5 = (12*(yf-y0)-(6*y_dotf+6*y_dot0)*tf-(y_ddot0-y_ddotf)*tf^2) / (2*tf^5);
    y = b0 + b1 * (t-40) + b2 * (t-40)^2 + b3 * (t-40)^3 + b4 * (t-40)^4 + b5 * (t-40)^5;

    z0 = 0.5; zf = z0 - 0.4; z_dot0 = 0; z_dotf = 0; z_ddot0 = 0; z_ddotf = 0;
    c0 = z0; c1 = z_dot0; c2 = z_ddot0 / 2;
    c3 = (20*(zf-z0)-(8*z_dotf+12*z_dot0)*tf-(3*z_ddot0-z_ddotf)*tf^2) / (2*tf^3);
    c4 = (30*(z0-zf)+(14*z_dotf+16*z_dot0)*tf+(3*z_ddot0-2*z_ddotf)*tf^2) / (2*tf^4);
    c5 = (12*(zf-z0)-(6*z_dotf+6*z_dot0)*tf-(z_ddot0-z_ddotf)*tf^2) / (2*tf^5);
    z = c0 + c1 * (t-ts) + c2 * (t-ts)^2 + c3 * (t-ts)^3 + c4 * (t-ts)^4 + c5 * (t-ts)^5;
    
    Xd = [x y z]';
else
    x = 0.5 + 0.1*sin(phi);
    y = 0.3 + 0.1*cos(phi);
    z = 0.1;
    
    Xd = [x y z]';
end
end

== matlab function TDE_with_NPD_ARAS/Forward Kinematics1 ==
  data: Jacobian output; Theta input; X output; L0 input
function [Jacobian, X] = fcn(Theta, L0)

a = 1.00;% + 0.05;
b = 1.00;% - 0.05;
c = 1.00;% - 0.05;
r = 0.03;% + 0.005;


L = [r * Theta(1) + L0(1)
     r * Theta(2) + L0(2)
     r * Theta(3) + L0(3)
     r * Theta(4) + L0(4)];

x = (L(2)^2 - L(3)^2 + a^2) / (2*a);
y = (L(1)^2 - L(2)^2 + b^2) / (2*b);
z = c - sqrt(L(1)^2 - x^2 - y^2);
X = [x y z]';

Jacobian = [(X(1)-0)/L(1)    (X(2)-0)/L(1)   (X(3)-c)/L(1)
            (X(1)-0)/L(2)    (X(2)-b)/L(2)   (X(3)-c)/L(2)
            (X(1)-a)/L(3)    (X(2)-b)/L(3)   (X(3)-c)/L(3)
            (X(1)-a)/L(4)    (X(2)-0)/L(4)   (X(3)-c)/L(4)];
end
